simulink model "model_kf"  (R2016b)
settings: Solver=FixedStepAuto  StartTime=0.0  StopTime=30  FixedStep=Ts  RelTol=1e-3  EnableMultiTasking=on
values from neighbouring files (symbols this model uses):
  C = [eye(3),zeros(3,9);zeros(3,6),eye(3),zeros(3,3);zeros(3,9),eye(3)]    [model_script.m]
  g = 9.81    [model_script.m]
  I = diag([Ixx;Iyy;Izz])    [model_script.m]
  M = 0.487    [model_script.m]
  mean_att = zeros(3,1)    [model_script.m]
  mean_av = zeros(3,1)    [model_script.m]
  mean_pos = zeros(3,1)    [model_script.m]
  Q = diag([1e-5,1e-5,1e-5,1e-7,1e-7,1e-4,ones(1,2)*2e-7,6e-7,ones(1,3)*1e-7])    [model_script.m]
  R = diag(var)    [model_script.m]
  T_att = 1/200    (= 0.005)    [model_script.m]
  T_xy = 1/10    (= 0.1)    [model_script.m]
  T_yaw = 1/100    (= 0.01)    [model_script.m]
  T_z = 1/25    (= 0.04)    [model_script.m]
  Ts = 1/400    (= 0.0025)    [model_script.m]
  var_att = [9.44454290406988e-06 1.41319492944844e-05 0.000590278082576831]'    [model_script.m]
  var_av = [8.38442613623844e-07 9.65548247114005e-07 1.06378940883219e-06]'    [model_script.m]
  var_pos = ones(3,1)*0.00219628793119666    [model_script.m]
undefined symbols (not defined in the file or in its folder): A, B, sigbuilder_block
libraries: aerolibutil x2, simulink x1
settings Model: PauseTimes=0.275  Creator=Patrick  LastModifiedBy=Patrick
settings OptimizationCC: LifeSpan=inf
settings DebuggingCC: SFUnexpectedBacktrackingDiag=warning  SFNoUnconditionalDefaultTransitionDiag=warning  SFExecutionAtInitializationDiag=none
settings GRTTargetCC: TargetLangStandard=C89/C90 (ANSI)  GeneratePreprocessorConditionals=Disable all
settings ConfigComp: CovMetricSettings=dw  CovHtmlReporting=on  CovSaveCumulativeToWorkspaceVar=on  CovSaveSingleToWorkspaceVar=on  CovExternalEMLEnable=off

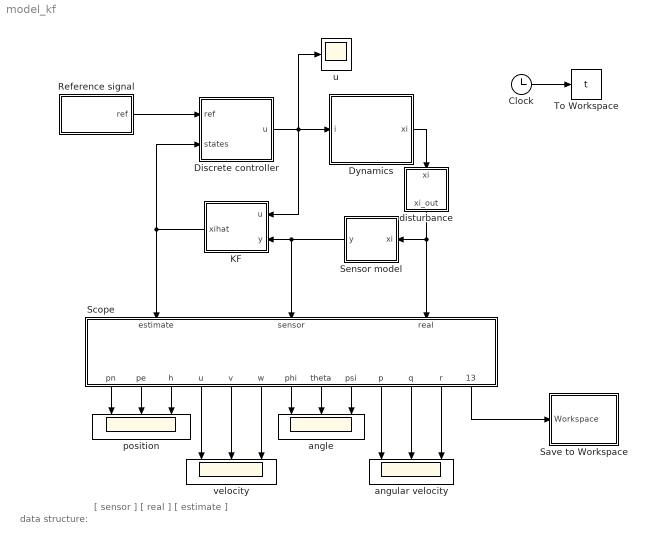
== system model_kf ==
  note: data structure:
  note: [ sensor   	]
      | [ real		]
      | [ estimate	]
  Clock : Clock
  Discrete controller : Subsystem
  Dynamics : Subsystem
  KF : Subsystem
  Reference signal : Subsystem
  Save to Workspace : Subsystem
  Scope : Subsystem
  Sensor model : Subsystem
  To Workspace : ToWorkspace  VariableName=t  SampleTime=-1
      settings: Decimation=10
  angle : Scope  NumInputPorts=3
  angular velocity : Scope  NumInputPorts=3
  disturbance : Subsystem
  position : Scope  NumInputPorts=3
  u : Scope
  velocity : Scope  NumInputPorts=3
  wires:
  Reference signal/1(ref) -> Discrete controller/1(ref)
  Scope/2(pe) -> position/2
  Scope/10(p) -> angular velocity/1
  Scope/6(w) -> velocity/3
  Scope/5(v) -> velocity/2
  Scope/1(pn) -> position/1
  Scope/8(theta) -> angle/2
  Scope/9(psi) -> angle/3
  Scope/4(u) -> velocity/1
  Scope/11(q) -> angular velocity/2
  Scope/12(r) -> angular velocity/3
  Scope/7(phi) -> angle/1
  Scope/3(h) -> position/3
  Dynamics/1(xi) -> disturbance/1(xi)
  KF/1(xihat) -> Discrete controller/2(states), Scope/1(estimate)
  Scope/13(Workspace) -> Save to Workspace/1(Workspace)
  Sensor model/1(y) -> Scope/2(sensor), KF/2(y)
  Discrete controller/1(u) -> KF/1(u), u/1, Dynamics/1(i)
  Clock/1 -> To Workspace/1
  disturbance/1(xi_out) -> Scope/3(real), Sensor model/1(xi)

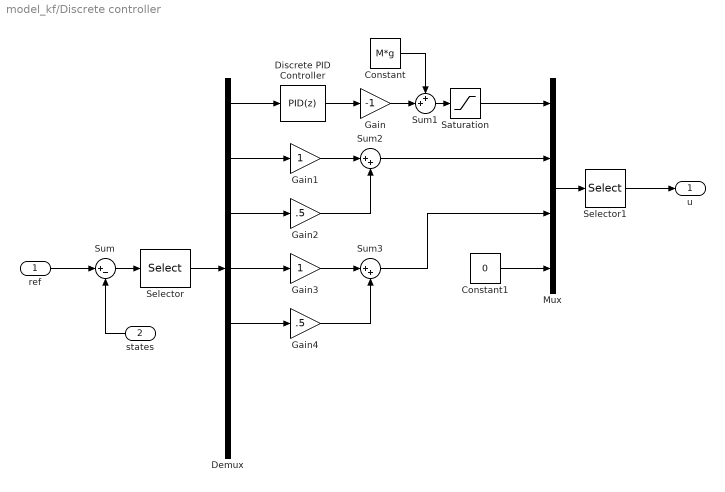
== system model_kf/Discrete controller ==
  ref : Inport
  states : Inport  Port=2
  Constant : Constant  Value=M*g
  Constant1 : Constant  Value=0
  Demux : Demux  Outputs=7
  Discrete PID Controller : simulink/Continuous/PID Controller  Controller=PID  TimeDomain=Discrete-time  SampleTime=-1  IntegratorMethod=Forward Euler  FilterMethod=Forward Euler  Form=Parallel  UseFilter=on  ControllerParametersSource=internal  P=2  I=0  D=1  N=100  InitialConditionSource=internal  InitialConditionForIntegrator=0  InitialConditionForFilter=0  ExternalReset=none  LimitOutput=off  UpperSaturationLimit=inf  LowerSaturationLimit=-inf  LinearizeAsGain=off  AntiWindupMode=none  Kb=1  TrackingMode=off  Kt=1  PParamMin=[]  PParamMax=[]  IParamMin=[]  IParamMax=[]  DParamMin=[]  DParamMax=[]  NParamMin=[]  NParamMax=[]  KbParamMin=[]  KbParamMax=[]  KtParamMin=[]  KtParamMax=[]  POutMin=[]  POutMax=[]  IOutMin=[]  IOutMax=[]  DOutMin=[]  DOutMax=[]  NOutMin=[]  NOutMax=[]  KbOutMin=[]  KbOutMax=[]  KtOutMin=[]  KtOutMax=[]  IntegratorOutMin=[]  IntegratorOutMax=[]  FilterOutMin=[]  FilterOutMax=[]  SumOutMin=[]  SumOutMax=[]  SumI1OutMin=[]  SumI1OutMax=[]  SumI2OutMin=[]  SumI2OutMax=[]  SumI3OutMin=[]  SumI3OutMax=[]  SumDOutMin=[]  SumDOutMax=[]  SaturationOutMin=[]  SaturationOutMax=[]  IntegratorContinuousStateAttributes=''  IntegratorStateMustResolveToSignalObject=off  IntegratorRTWStateStorageClass=Auto  FilterContinuousStateAttributes=''  FilterStateMustResolveToSignalObject=off  FilterRTWStateStorageClass=Auto  DifferentiatorICPrevScaledInput=0  DifferentiatorOutMin=[]  DifferentiatorOutMax=[]
  Gain : Gain  Gain=-1
  Gain1 : Gain
  Gain2 : Gain  Gain=.5
  Gain3 : Gain
  Gain4 : Gain  Gain=.5
  Mux : Mux
  Saturation : Saturate  UpperLimit=10  LowerLimit=-10
  Selector : Selector  InputPortWidth=12  IndexOptions=Index vector (dialog)  Indices="[3 7  10 8 11 9 12]"  OutputSizes=1
  Selector1 : Selector  InputPortWidth=4  IndexOptions=Index vector (dialog)  Indices=[2 3 4 1]  OutputSizes=1
  Sum : Sum  Inputs=|+-
  Sum1 : Sum  Inputs=++|
  Sum2 : Sum  Inputs=|++
  Sum3 : Sum  Inputs=|++
  u : Outport
  wires:
  Demux/1 -> Discrete PID Controller/1
  ref/1 -> Sum/1
  states/1 -> Sum/2
  Discrete PID Controller/1 -> Gain/1
  Sum/1 -> Selector/1
  Selector/1 -> Demux/1
  Sum1/1 -> Saturation/1
  Constant/1 -> Sum1/1
  Gain/1 -> Sum1/2
  Demux/2 -> Gain1/1
  Demux/3 -> Gain2/1
  Gain1/1 -> Sum2/1
  Gain2/1 -> Sum2/2
  Saturation/1 -> Mux/1
  Sum2/1 -> Mux/2
  Demux/4 -> Gain3/1
  Demux/5 -> Gain4/1
  Gain3/1 -> Sum3/1
  Gain4/1 -> Sum3/2
  Sum3/1 -> Mux/3
  Mux/1 -> Selector1/1
  Selector1/1 -> u/1
  Constant1/1 -> Mux/4

== system model_kf/Dynamics ==
  i : Inport
  Dynamics : Subsystem
  Mux : Mux
  xi : Outport
  wires:
  Mux/1 -> xi/1
  i/1 -> Dynamics/1(i)
  Dynamics/1(x y z) -> Mux/1
  Dynamics/2(u v w) -> Mux/2
  Dynamics/3(phi theta psi) -> Mux/3
  Dynamics/4(p q r) -> Mux/4

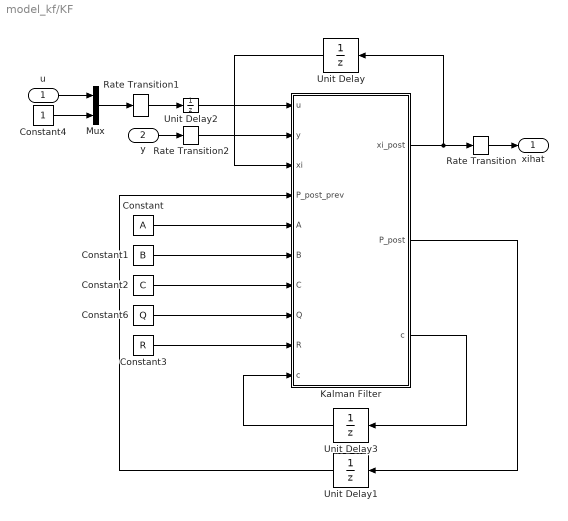
== system model_kf/KF ==
  u : Inport
  y : Inport  Port=2
  Constant : Constant  Value=A
  Constant1 : Constant  Value=B
  Constant2 : Constant  Value=C
  Constant3 : Constant  Value=R
  Constant4 : Constant
  Constant6 : Constant  Value=Q
  Kalman Filter : MATLAB Function  TreatAsAtomicUnit=on
  Mux : Mux  Inputs=2
  Rate Transition : RateTransition  OutPortSampleTime=Ts
  Rate Transition1 : RateTransition  OutPortSampleTime=Ts
  Rate Transition2 : RateTransition  OutPortSampleTime=Ts
  Unit Delay : UnitDelay  InitialCondition=[0;0;0;0;0;0;0;0;0;0;0;0]  SampleTime=Ts
  Unit Delay1 : UnitDelay  InitialCondition=zeros(12,12)  SampleTime=Ts
  Unit Delay2 : UnitDelay  InitialCondition=[0;0;0;0;1]  SampleTime=Ts
  Unit Delay3 : UnitDelay  SampleTime=-1
  xihat : Outport
  wires:
  Constant/1 -> Kalman Filter/5(A)
  Constant1/1 -> Kalman Filter/6(B)
  Constant2/1 -> Kalman Filter/7(C)
  Constant6/1 -> Kalman Filter/8(Q)
  y/1 -> Rate Transition2/1
  Unit Delay/1 -> Kalman Filter/3(xi)
  Unit Delay1/1 -> Kalman Filter/4(P_post_prev)
  Kalman Filter/1(xi_post) -> Unit Delay/1, Rate Transition/1
  Kalman Filter/2(P_post) -> Unit Delay1/1
  Rate Transition2/1 -> Kalman Filter/2(y)
  Unit Delay2/1 -> Kalman Filter/1(u)
  Constant3/1 -> Kalman Filter/9(R)
  Mux/1 -> Rate Transition1/1
  u/1 -> Mux/1
  Constant4/1 -> Mux/2
  Rate Transition1/1 -> Unit Delay2/1
  Rate Transition/1 -> xihat/1
  Unit Delay3/1 -> Kalman Filter/10("c ")
  Kalman Filter/3(c) -> Unit Delay3/1

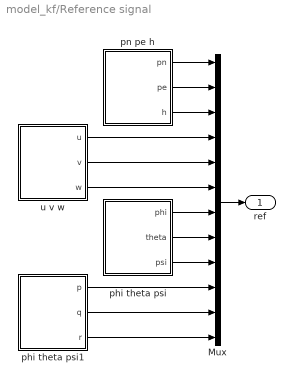
== system model_kf/Reference signal ==
  Mux : Mux  Inputs=12
  phi theta psi : Subsystem
  phi theta psi1 : Subsystem
  pn pe h : Subsystem
  u v w : Subsystem
  ref : Outport
  wires:
  pn pe h/1(pn) -> Mux/1
  pn pe h/2(pe) -> Mux/2
  pn pe h/3(h) -> Mux/3
  u v w/1(u) -> Mux/4
  u v w/2(v) -> Mux/5
  u v w/3(w) -> Mux/6
  phi theta psi/1(phi) -> Mux/7
  phi theta psi/2(theta) -> Mux/8
  phi theta psi/3(psi) -> Mux/9
  phi theta psi1/1(p) -> Mux/10
  phi theta psi1/2(q) -> Mux/11
  phi theta psi1/3(r) -> Mux/12
  Mux/1 -> ref/1

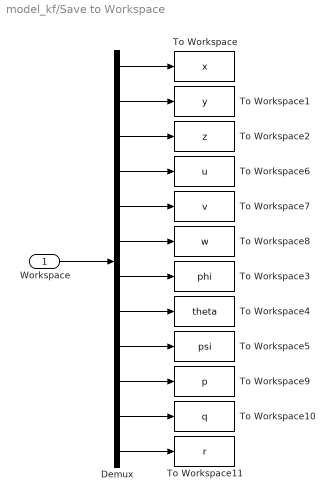
== system model_kf/Save to Workspace ==
  Workspace : Inport
  Demux : Demux  Outputs=12
  To Workspace : ToWorkspace  VariableName=x  SampleTime=-1
      settings: Decimation=10
  To Workspace1 : ToWorkspace  VariableName=y  SampleTime=-1
      settings: Decimation=10
  To Workspace10 : ToWorkspace  VariableName=q  SampleTime=-1
      settings: Decimation=10
  To Workspace11 : ToWorkspace  VariableName=r  SampleTime=-1
      settings: Decimation=10
  To Workspace2 : ToWorkspace  VariableName=z  SampleTime=-1
      settings: Decimation=10
  To Workspace3 : ToWorkspace  VariableName=phi  SampleTime=-1
      settings: Decimation=10
  To Workspace4 : ToWorkspace  VariableName=theta  SampleTime=-1
      settings: Decimation=10
  To Workspace5 : ToWorkspace  VariableName=psi  SampleTime=-1
      settings: Decimation=10
  To Workspace6 : ToWorkspace  VariableName=u  SampleTime=-1
      settings: Decimation=10
  To Workspace7 : ToWorkspace  VariableName=v  SampleTime=-1
      settings: Decimation=10
  To Workspace8 : ToWorkspace  VariableName=w  SampleTime=-1
      settings: Decimation=10
  To Workspace9 : ToWorkspace  VariableName=p  SampleTime=-1
      settings: Decimation=10
  wires:
  Workspace/1 -> Demux/1
  Demux/1 -> To Workspace/1
  Demux/2 -> To Workspace1/1
  Demux/3 -> To Workspace2/1
  Demux/4 -> To Workspace6/1
  Demux/5 -> To Workspace7/1
  Demux/6 -> To Workspace8/1
  Demux/7 -> To Workspace3/1
  Demux/8 -> To Workspace4/1
  Demux/10 -> To Workspace9/1
  Demux/9 -> To Workspace5/1
  Demux/11 -> To Workspace10/1
  Demux/12 -> To Workspace11/1

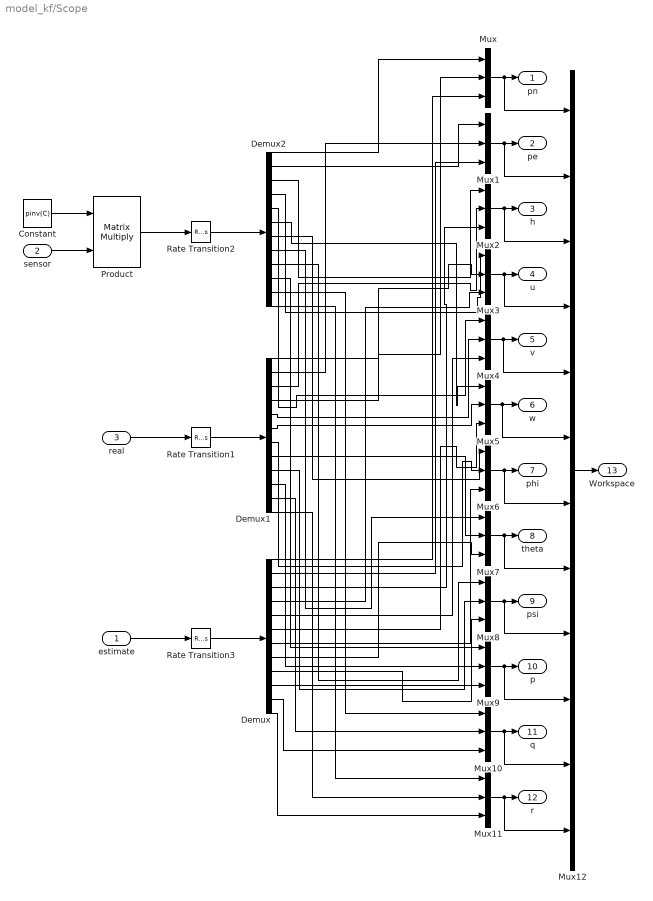
== system model_kf/Scope ==
  estimate : Inport
  sensor : Inport  Port=2
  real : Inport  Port=3
  Constant : Constant  Value=pinv(C)
  Demux : Demux  Outputs=12
  Demux1 : Demux  Outputs=12
  Demux2 : Demux  Outputs=12
  Mux{,1..11} (12 alike) : Mux  Inputs=3
  Mux12 : Mux  Inputs=12
  Product : Product  Multiplication=Matrix(*)
  Rate Transition1 : RateTransition  OutPortSampleTime=Ts
  Rate Transition2 : RateTransition  OutPortSampleTime=Ts
  Rate Transition3 : RateTransition  OutPortSampleTime=Ts
  pn : Outport
  pe : Outport  Port=2
  h : Outport  Port=3
  u : Outport  Port=4
  v : Outport  Port=5
  w : Outport  Port=6
  phi : Outport  Port=7
  theta : Outport  Port=8
  psi : Outport  Port=9
  p : Outport  Port=10
  q : Outport  Port=11
  r : Outport  Port=12
  Workspace : Outport  Port=13
  wires:
  Demux2/1 -> Mux/1
  Demux1/1 -> Mux/2
  Demux/1 -> Mux/3
  Demux2/2 -> Mux1/1
  Demux1/2 -> Mux1/2
  Demux/2 -> Mux1/3
  Demux2/3 -> Mux2/1
  Demux1/3 -> Mux2/2
  Demux/3 -> Mux2/3
  Mux/1 -> Mux12/1, pn/1
  Mux1/1 -> Mux12/2, pe/1
  Demux2/4 -> Mux3/1
  Demux1/4 -> Mux3/2
  Demux/4 -> Mux3/3
  Mux3/1 -> Mux12/4, u/1
  Demux2/5 -> Mux4/1
  Demux1/5 -> Mux4/2
  Demux/5 -> Mux4/3
  Mux4/1 -> Mux12/5, v/1
  Demux2/6 -> Mux5/1
  Demux1/6 -> Mux5/2
  Demux/6 -> Mux5/3
  Mux5/1 -> Mux12/6, w/1
  Mux6/1 -> Mux12/7, phi/1
  Demux2/7 -> Mux6/1
  Demux1/7 -> Mux6/2
  Demux/7 -> Mux6/3
  Mux7/1 -> Mux12/8, theta/1
  Demux2/8 -> Mux7/1
  Demux1/8 -> Mux7/2
  Demux/8 -> Mux7/3
  Mux8/1 -> Mux12/9, psi/1
  Demux2/9 -> Mux8/1
  Demux1/9 -> Mux8/2
  Demux/9 -> Mux8/3
  Mux9/1 -> Mux12/10, p/1
  Mux10/1 -> Mux12/11, q/1
  Mux11/1 -> Mux12/12, r/1
  Demux2/10 -> Mux9/1
  Demux1/10 -> Mux9/2
  Demux/10 -> Mux9/3
  Demux2/11 -> Mux10/1
  Demux1/11 -> Mux10/2
  Demux/11 -> Mux10/3
  Demux2/12 -> Mux11/1
  Demux1/12 -> Mux11/2
  Demux/12 -> Mux11/3
  estimate/1 -> Rate Transition3/1
  real/1 -> Rate Transition1/1
  Mux2/1 -> Mux12/3, h/1
  Mux12/1 -> Workspace/1
  sensor/1 -> Product/2
  Product/1 -> Rate Transition2/1
  Constant/1 -> Product/1
  Rate Transition2/1 -> Demux2/1
  Rate Transition1/1 -> Demux1/1
  Rate Transition3/1 -> Demux/1

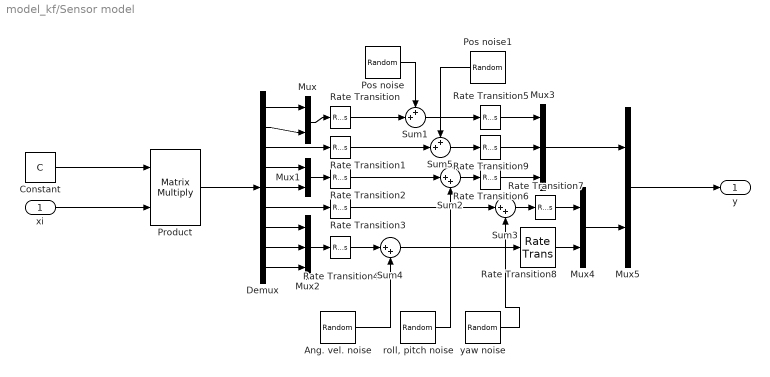
== system model_kf/Sensor model ==
  xi : Inport
  Ang. vel. noise : RandomNumber  Mean=mean_av  Variance=var_av  Seed=[7;8;9]  SampleTime=T_yaw  VectorParams1D=off
  Constant : Constant  Value=C
  Demux : Demux  Outputs=9
  Mux{,1,4..5} (4 alike) : Mux  Inputs=2
  Mux2 : Mux  Inputs=3
  Mux3 : Mux  Inputs=3
  Pos noise : RandomNumber  Mean=mean_pos(1:2)  Variance=var_pos(1:2)  Seed=[1;2]  SampleTime=T_xy  VectorParams1D=off
  Pos noise1 : RandomNumber  Mean=mean_pos(3)  Variance=var_pos(3)  Seed=3  SampleTime=T_z  VectorParams1D=off
  Product : Product  Multiplication=Matrix(*)
  Rate Transition : RateTransition  OutPortSampleTime=T_xy
  Rate Transition1 : RateTransition  OutPortSampleTime=T_z
  Rate Transition2 : RateTransition  OutPortSampleTime=T_att
  Rate Transition3 : RateTransition  OutPortSampleTime=T_yaw
  Rate Transition4 : RateTransition  OutPortSampleTime=T_yaw
  Rate Transition{5..9} (5 alike) : RateTransition  OutPortSampleTime=Ts
  Sum1 : Sum  Inputs=++|
  Sum2 : Sum  Inputs=|++
  Sum3 : Sum  Inputs=|++
  Sum4 : Sum  Inputs=|++
  Sum5 : Sum  Inputs=++|
  "roll, pitch noise" : RandomNumber  Mean=mean_att(1:2)  Variance=var_att(1:2)  Seed=[4;5]  SampleTime=T_att  VectorParams1D=off
  yaw noise : RandomNumber  Mean=mean_att(3,1)  Variance=var_att(3,1)  Seed=6  SampleTime=T_yaw  VectorParams1D=off
  y : Outport
  wires:
  xi/1 -> Product/2
  Constant/1 -> Product/1
  "roll, pitch noise"/1 -> Sum2/2
  yaw noise/1 -> Sum3/2
  Ang. vel. noise/1 -> Sum4/2
  Product/1 -> Demux/1
  Demux/3 -> Rate Transition1/1
  Demux/2 -> Mux/2
  Demux/1 -> Mux/1
  Demux/4 -> Mux1/1
  Demux/5 -> Mux1/2
  Pos noise/1 -> Sum1/1
  Mux/1 -> Rate Transition/1
  Mux1/1 -> Rate Transition2/1
  Demux/6 -> Rate Transition3/1
  Demux/7 -> Mux2/1
  Demux/8 -> Mux2/2
  Demux/9 -> Mux2/3
  Mux2/1 -> Rate Transition4/1
  Sum1/1 -> Rate Transition5/1
  Sum2/1 -> Rate Transition6/1
  Sum3/1 -> Rate Transition7/1
  Sum4/1 -> Rate Transition8/1
  Mux3/1 -> Mux5/1
  Mux4/1 -> Mux5/2
  Rate Transition/1 -> Sum1/2
  Rate Transition2/1 -> Sum2/1
  Rate Transition3/1 -> Sum3/1
  Rate Transition4/1 -> Sum4/1
  Mux5/1 -> y/1
  Rate Transition5/1 -> Mux3/1
  Rate Transition7/1 -> Mux4/1
  Rate Transition8/1 -> Mux4/2
  Rate Transition6/1 -> Mux3/3
  Pos noise1/1 -> Sum5/1
  Sum5/1 -> Rate Transition9/1
  Rate Transition1/1 -> Sum5/2
  Rate Transition9/1 -> Mux3/2

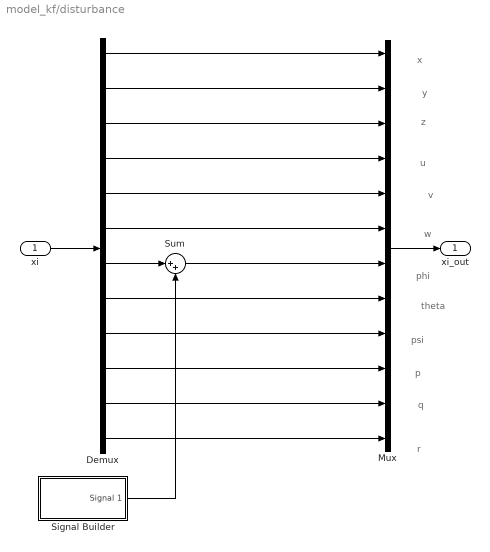
== system model_kf/disturbance ==
  note: r
  note: q
  note: p
  note: psi
  note: theta
  note: phi
  note: w
  note: v
  note: u
  note: z
  note: y
  note: x
  xi : Inport
  Demux : Demux  Outputs=12
  Mux : Mux  Inputs=12
  Signal Builder : Subsystem  Tag=STV Subsys  LoadFcn=sigbuilder_block('load');  StartFcn=sigbuilder_block('start');  StopFcn=sigbuilder_block('stop');  ClipboardFcn=sigbuilder_block('clipboard');  mask(Sigbuilder block){tuvar=[0:10]}
      mask help: Simulink:masks:SigbuilderBlock_MD
      mask init:
      | if ~strcmp(get_param(bdroot(gcbh),'SimulationStatus'),'stopped') tuvar = sigbuilder_block('maskInit'); end
      settings: CopyFcn=sigbuilder_block('copy');  DeleteFcn=sigbuilder_block('delete');  ModelCloseFcn=sigbuilder_block('modelClose');  PreSaveFcn=sigbuilder_block('preSave');  PauseFcn=sigbuilder_block('pause');  ContinueFcn=sigbuilder_block('continue');  NameChangeFcn=sigbuilder_block('namechange');  OpenFcn=sigbuilder_block('open',[437.6 199.2 550.4 400 ]);  CloseFcn=sigbuilder_block('close');
      mask Display: plot(0, 0, 100, 100,[2, 2, 32, 32, 2], [68, 8, 8, 68, 68],[32, 2], [38, 38], [32, 19, 2],[53, 60, 44], [32, 17, 17, 2],[16, 16, 31, 31]);txt = getActiveGroup(gcbh);text(2, 100, txt,'verticalAlignment', 'top');
  Sum : Sum  Inputs=|++
  xi_out : Outport
  wires:
  xi/1 -> Demux/1
  Demux/12 -> Mux/12
  Demux/11 -> Mux/11
  Demux/1 -> Mux/1
  Demux/2 -> Mux/2
  Demux/3 -> Mux/3
  Demux/4 -> Mux/4
  Demux/5 -> Mux/5
  Demux/6 -> Mux/6
  Demux/8 -> Mux/8
  Demux/9 -> Mux/9
  Demux/10 -> Mux/10
  Mux/1 -> xi_out/1
  Demux/7 -> Sum/1
  Sum/1 -> Mux/7
  Signal Builder/1(Signal 1) -> Sum/2

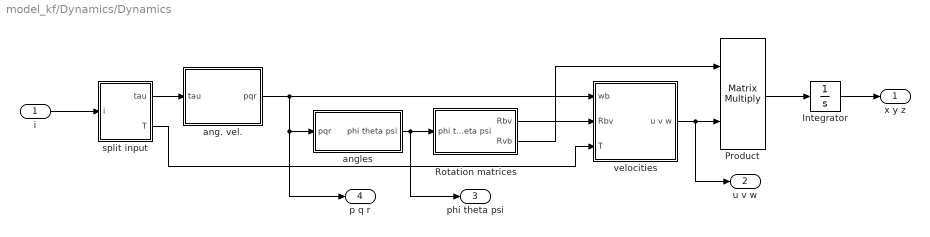
== system model_kf/Dynamics/Dynamics ==
  i : Inport
  Integrator : Integrator  InitialCondition=[0;0;0]
  Product : Product  Multiplication=Matrix(*)
  Rotation matrices : Subsystem
  ang. vel. : Subsystem
  angles : Subsystem
  split input : Subsystem
  velocities : Subsystem
  x y z : Outport
  u v w : Outport  Port=2
  phi theta psi : Outport  Port=3
  p q r : Outport  Port=4
  wires:
  Product/1 -> Integrator/1
  Rotation matrices/2(Rvb) -> Product/1
  ang. vel./1(pqr) -> angles/1(pqr), p q r/1, velocities/1(wb)
  angles/1(phi theta psi) -> Rotation matrices/1(phi theta psi), phi theta psi/1
  velocities/1(u v w) -> u v w/1, Product/2
  Rotation matrices/1(Rbv) -> velocities/2(Rbv)
  i/1 -> split input/1(i)
  split input/1(tau) -> ang. vel./1(tau)
  split input/2(T) -> velocities/3(T)
  Integrator/1 -> x y z/1

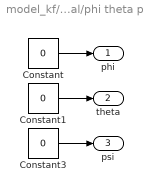
== system model_kf/Reference signal/phi theta psi ==
  Constant : Constant  Value=0
  Constant1 : Constant  Value=0
  Constant3 : Constant  Value=0
  phi : Outport
  theta : Outport  Port=2
  psi : Outport  Port=3
  wires:
  Constant3/1 -> psi/1
  Constant1/1 -> theta/1
  Constant/1 -> phi/1

== system model_kf/Reference signal/phi theta psi1 ==
  Constant1 : Constant  Value=0
  Constant2 : Constant  Value=0
  Constant3 : Constant  Value=0
  p : Outport
  q : Outport  Port=2
  r : Outport  Port=3
  wires:
  Constant1/1 -> p/1
  Constant2/1 -> q/1
  Constant3/1 -> r/1

== system model_kf/Reference signal/pn pe h ==
  Constant : Constant  Value=-0.8
  Step : Step  Time=5  SampleTime=0
  Step1 : Step  Time=5  SampleTime=0
  pn : Outport
  pe : Outport  Port=2
  h : Outport  Port=3
  wires:
  Constant/1 -> h/1
  Step1/1 -> pe/1
  Step/1 -> pn/1

== system model_kf/Reference signal/u v w ==
  Constant1 : Constant  Value=0
  Constant2 : Constant  Value=0
  Constant3 : Constant  Value=0
  u : Outport
  v : Outport  Port=2
  w : Outport  Port=3
  wires:
  Constant3/1 -> w/1
  Constant1/1 -> u/1
  Constant2/1 -> v/1

== system model_kf/disturbance/Signal Builder ==
  Demux : Demux  Tag=STV Demux  Outputs=1
  FromWs : FromWorkspace  Tag=STV FromWs  VariableName=tuvar  SampleTime=0
      SigBuilderData=|
      | common.afterFinalStr = 'Extrapolate'
      | common.sampleTime = 0
      | dataSet.timeRange = [0 30]
      | dataSet.name = 'Group 1'
      | sbobj.Groups.Name = 'Group 1'
      | sbobj.Groups.Signals.Name = 'Signal 1'
      | sbobj.Groups.Signals.XData = [0 5 5 6 6 30]
      | sbobj.Groups.Signals.YData = [0 0 0.02 0.02 0 0]
      | sbobj.Groups.TimeRange = [0 30]
  Signal 1 : Outport  Tag=STV Outport
  wires:
  Demux/1 -> Signal 1/1
  FromWs/1 -> Demux/1

== system model_kf/Dynamics/Dynamics/Rotation matrices ==
  phi theta psi : Inport
  Rotm in euler : MATLAB Function  TreatAsAtomicUnit=on
  Transpose : Math  Operator=transpose  SaturateOnIntegerOverflow=on
  Rbv : Outport
  Rvb : Outport  Port=2
  wires:
  phi theta psi/1 -> Rotm in euler/1(alpha)
  Rotm in euler/1(Rbv) -> Rbv/1, Transpose/1
  Transpose/1 -> Rvb/1

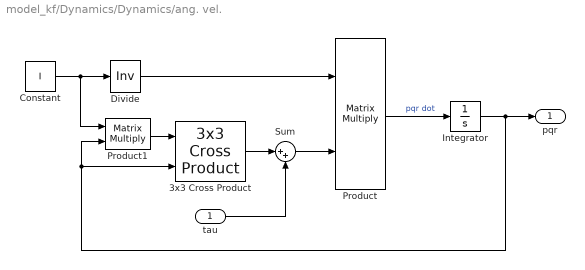
== system model_kf/Dynamics/Dynamics/ang. vel. ==
  tau : Inport
  3x3 Cross Product : aerolibutil/3x3 Cross Product
  Constant : Constant  Value=I
  Divide : Product  Inputs=/  Multiplication=Matrix(*)
  Integrator : Integrator
  Product : Product  Multiplication=Matrix(*)
  Product1 : Product  Multiplication=Matrix(*)
  Sum : Sum  Inputs=|++
  pqr : Outport
  wires:
  Constant/1 -> Product1/1, Divide/1
  Sum/1 -> Product/2
  tau/1 -> Sum/2
  3x3 Cross Product/1 -> Sum/1
  Product1/1 -> 3x3 Cross Product/1
  Divide/1 -> Product/1
  Integrator/1 -> pqr/1, 3x3 Cross Product/2, Product1/2
  Product/1 -> Integrator/1  "pqr dot"

== system model_kf/Dynamics/Dynamics/angles ==
  pqr : Inport
  Integrator : Integrator  InitialCondition=[0;0;0]
  MATLAB Function : MATLAB Function  TreatAsAtomicUnit=on
  Product : Product  Multiplication=Matrix(*)
  phi theta psi : Outport
  wires:
  MATLAB Function/1(E) -> Product/1
  pqr/1 -> Product/2
  Product/1 -> Integrator/1  "phi theta psi dot"
  Integrator/1 -> phi theta psi/1, MATLAB Function/1(alpha)

== system model_kf/Dynamics/Dynamics/split input ==
  i : Inport
  Demux : Demux
  Mux : Mux  Inputs=3
  tau : Outport
  T : Outport  Port=2
  wires:
  Demux/2 -> Mux/2
  Demux/3 -> Mux/3
  i/1 -> Demux/1
  Mux/1 -> tau/1
  Demux/4 -> T/1
  Demux/1 -> Mux/1

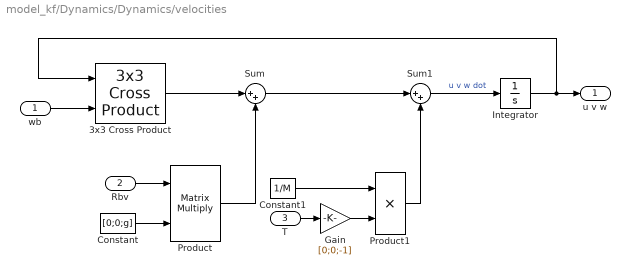
== system model_kf/Dynamics/Dynamics/velocities ==
  wb : Inport
  Rbv : Inport  Port=2
  T : Inport  Port=3
  3x3 Cross Product : aerolibutil/3x3 Cross Product
  Constant : Constant  Value=[0;0;g]
  Constant1 : Constant  Value=1/M
  Gain : Gain  Gain=[0;0;-1]
  Integrator : Integrator
  Product : Product  Multiplication=Matrix(*)
  Product1 : Product
  Sum : Sum  Inputs=|++
  Sum1 : Sum  Inputs=|++
  u v w : Outport
  wires:
  3x3 Cross Product/1 -> Sum/1
  wb/1 -> 3x3 Cross Product/2
  Product/1 -> Sum/2
  Rbv/1 -> Product/1
  Constant/1 -> Product/2
  Sum/1 -> Sum1/1
  Product1/1 -> Sum1/2
  Constant1/1 -> Product1/1
  T/1 -> Gain/1
  Sum1/1 -> Integrator/1  "u v w dot"
  Integrator/1 -> 3x3 Cross Product/1, u v w/1
  Gain/1 -> Product1/2

== matlab function model_kf/KF/Kalman Filter ==
  data: u input; xi_post output; y input; xi input; P_post_prev input; A input; B input; C input; Q input; R input; P_post output; c input; c output
function [xi_post,P_post,c] = fcn(u,y,xi,P_post_prev,A,B,C,Q,R,c)
%% Prediction
x_prio = A*xi + B*u;
P_prio = A*P_post_prev*A'+Q;

%% Update
K = P_prio*C'/(C*P_prio*C'+R);

% Only update states where new sensor data is received
if mod(c,2) ~= 0
    K(:,4:5) = 0;
    K(:,7:9) = 0;
end
if mod(c,4) ~= 0
    K(:,6) = 0;
end
if mod(c,16) ~= 0
    K(:,3) = 0;
end
if mod(c,40) ~= 0
    K(:,1:2) = 0;
end
c = c+1;
if c == 80
    c = 0;
end

% Update states and covariance matrix
xi_post = x_prio + K*(y-C*x_prio);
P_post = (eye(size(P_prio,1))-K*C)*P_prio*(eye(size(P_prio,1))-K*C)'+K*R*K';

== matlab function model_kf/Dynamics/Dynamics/Rotation matrices/Rotm in euler ==
  data: alpha input; Rbv output
function Rbv = fcn(alpha)
Rbv = [1,0,0;0,cos(alpha(1)),sin(alpha(1));0,-sin(alpha(1)),cos(alpha(1))]*...
      [cos(alpha(2)),0,-sin(alpha(2));0,1,0;sin(alpha(2)),0,cos(alpha(2))]*...
      [cos(alpha(3)),sin(alpha(3)),0;-sin(alpha(3)),cos(alpha(3)),0;0,0,1];

== matlab function model_kf/Dynamics/Dynamics/angles/MATLAB Function ==
  data: alpha input; E output
function E = fcn(alpha)
E = [1, sin(alpha(1))*tan(alpha(2)),cos(alpha(1))*tan(alpha(2));...
     0,               cos(alpha(1)),             -sin(alpha(1));...
     0, sin(alpha(1))/cos(alpha(2)),cos(alpha(1))/cos(alpha(2))];
